simulink model "test_p"  (R2017b)
settings: Solver=VariableStepAuto  StartTime=0.0  StopTime=10.0  RelTol=1e-3
libraries: arduinolib x12
settings Model: Creator=HRUSHIKESH  LastModifiedBy=HRUSHIKESH

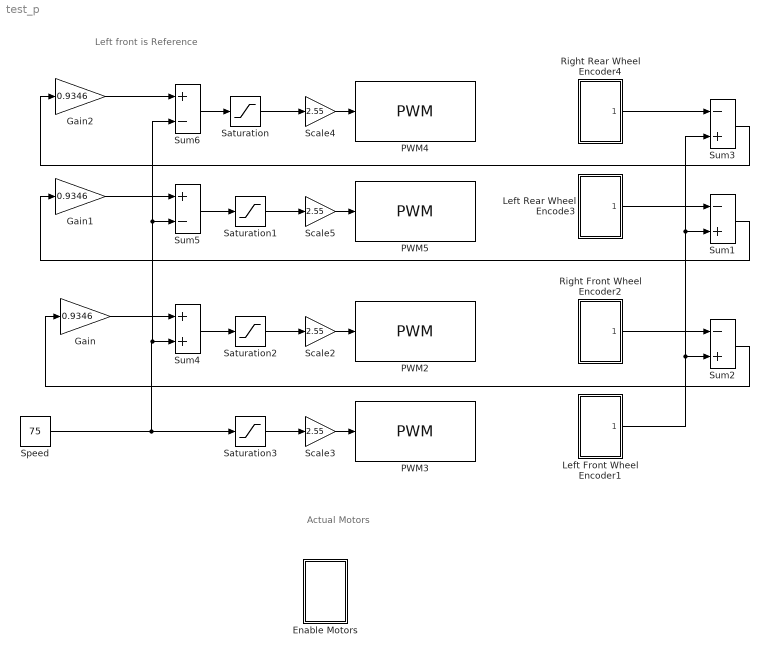
== system test_p ==
  note: Left front is Reference
  note: Actual
      | Motors
  Enable Motors : Subsystem
  Gain : Gain  Gain=0.9346  ParamDataTypeStr=single
  Gain1 : Gain  Gain=0.9346  ParamDataTypeStr=single
  Gain2 : Gain  Gain=0.9346  ParamDataTypeStr=single
  Left Front Wheel Encoder1 : Subsystem
  Left Rear Wheel Encode3 : Subsystem
  PWM2 : arduinolib/PWM  pinNumber=10  blockPlatform=arduino
  PWM3 : arduinolib/PWM  pinNumber=11  blockPlatform=arduino
  PWM4 : arduinolib/PWM  pinNumber=6  blockPlatform=arduino
  PWM5 : arduinolib/PWM  pinNumber=9  blockPlatform=arduino
  Right Front Wheel Encoder2 : Subsystem
  Right Rear Wheel Encoder4 : Subsystem
  Saturation{,1..3} (4 alike) : Saturate  UpperLimit=100  LowerLimit=0
      settings: AttributesFormatString=max = %<UpperLimit>\nmin = %<LowerLimit>
  Scale{2..5} (4 alike) : Gain  Gain=2.55
  Speed : Constant  Value=75  OutMin=0  OutMax=100  OutDataTypeStr=single  SampleTime=0.001
  Sum1 : Sum  Inputs=-+  OutDataTypeStr=Inherit: Same as first input
  Sum2 : Sum  Inputs=-+  OutDataTypeStr=Inherit: Same as first input
  Sum3 : Sum  Inputs=-+  OutDataTypeStr=Inherit: Same as first input
  Sum4 : Sum  OutDataTypeStr=Inherit: Same as first input
  Sum5 : Sum  Inputs=+-  OutDataTypeStr=Inherit: Same as first input
  Sum6 : Sum  Inputs=+-  OutDataTypeStr=Inherit: Same as first input
  wires:
  Scale2/1 -> PWM2/1
  Scale3/1 -> PWM3/1
  Right Rear Wheel Encoder4/1(Encoder) -> Sum3/1
  Scale4/1 -> PWM4/1
  Scale5/1 -> PWM5/1
  Sum3/1 -> Gain2/1
  Right Front Wheel Encoder2/1(Encoder) -> Sum2/1
  Left Rear Wheel Encode3/1(Encoder) -> Sum1/1
  Left Front Wheel Encoder1/1(Encoder) -> Sum3/2, Sum1/2, Sum2/2
  Saturation/1 -> Scale4/1
  Saturation1/1 -> Scale5/1
  Saturation2/1 -> Scale2/1
  Saturation3/1 -> Scale3/1
  Sum1/1 -> Gain1/1
  Sum2/1 -> Gain/1
  Sum6/1 -> Saturation/1
  Sum5/1 -> Saturation1/1
  Sum4/1 -> Saturation2/1
  Speed/1 -> Sum5/2, Sum6/2, Sum4/2, Saturation3/1
  Gain/1 -> Sum4/1
  Gain2/1 -> Sum6/1
  Gain1/1 -> Sum5/1

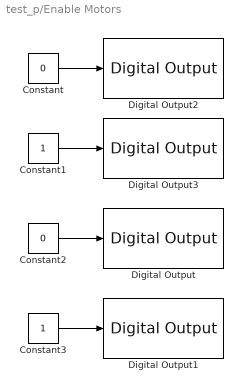
== system test_p/Enable Motors ==
  Constant : Constant  Value=0  OutDataTypeStr=boolean
  Constant1 : Constant  OutDataTypeStr=boolean
  Constant2 : Constant  Value=0  OutDataTypeStr=boolean
  Constant3 : Constant  OutDataTypeStr=boolean
  Digital Output : arduinolib/Digital Output  pinNumber=a1  blockPlatform=arduino
  Digital Output1 : arduinolib/Digital Output  pinNumber=a0  blockPlatform=arduino
  Digital Output2 : arduinolib/Digital Output  pinNumber=a3  blockPlatform=arduino
  Digital Output3 : arduinolib/Digital Output  pinNumber=a2  blockPlatform=arduino
  wires:
  Constant3/1 -> Digital Output1/1
  Constant2/1 -> Digital Output/1
  Constant/1 -> Digital Output2/1
  Constant1/1 -> Digital Output3/1

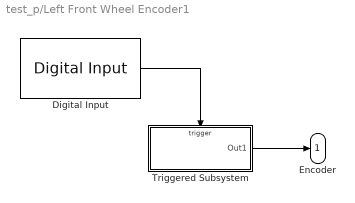
== system test_p/Left Front Wheel Encoder1 ==
  Digital Input : arduinolib/Digital Input  pinNumber=1  sampleTime=0.001  blockPlatform=arduino
      settings: SourceProductName=Simulink Support Package for Arduino Hardware
  Triggered Subsystem : Subsystem  TreatAsAtomicUnit=on
  Encoder : Outport
  wires:
  Triggered Subsystem/1(Out1) -> Encoder/1
  Digital Input/1 -> Triggered Subsystem/Trigger

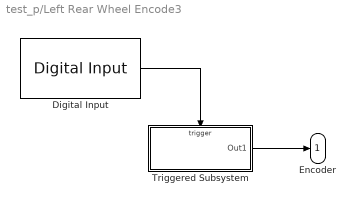
== system test_p/Left Rear Wheel Encode3 ==
  Digital Input : arduinolib/Digital Input  pinNumber=3  sampleTime=0.001  blockPlatform=arduino
      settings: SourceProductName=Simulink Support Package for Arduino Hardware
  Triggered Subsystem : Subsystem  TreatAsAtomicUnit=on
  Encoder : Outport
  wires:
  Triggered Subsystem/1(Out1) -> Encoder/1
  Digital Input/1 -> Triggered Subsystem/Trigger

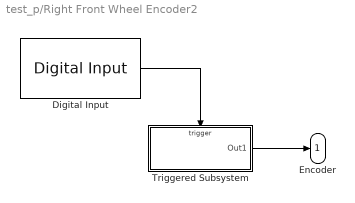
== system test_p/Right Front Wheel Encoder2 ==
  Digital Input : arduinolib/Digital Input  pinNumber=2  sampleTime=0.001  blockPlatform=arduino
      settings: SourceProductName=Simulink Support Package for Arduino Hardware
  Triggered Subsystem : Subsystem  TreatAsAtomicUnit=on
  Encoder : Outport
  wires:
  Digital Input/1 -> Triggered Subsystem/Trigger
  Triggered Subsystem/1(Out1) -> Encoder/1

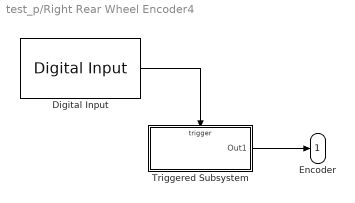
== system test_p/Right Rear Wheel Encoder4 ==
  Digital Input : arduinolib/Digital Input  pinNumber=4  sampleTime=0.001  blockPlatform=arduino
      settings: SourceProductName=Simulink Support Package for Arduino Hardware
  Triggered Subsystem : Subsystem  TreatAsAtomicUnit=on
  Encoder : Outport
  wires:
  Digital Input/1 -> Triggered Subsystem/Trigger
  Triggered Subsystem/1(Out1) -> Encoder/1

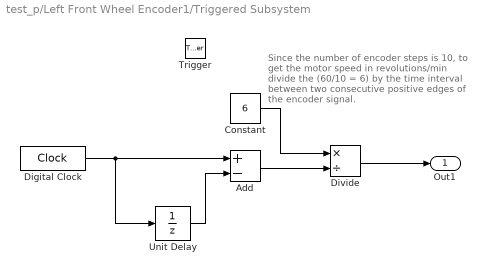
== system test_p/Left Front Wheel Encoder1/Triggered Subsystem ==
  note: Since the number of encoder steps is 10,
      | to get the motor speed in revolutions/min
      | divide the (60/10 = 6) by the time interval
      | between two consecutive positive edges
      | of the encoder signal.
  Trigger : TriggerPort  VariantControl=Variant
  Add : Sum  Inputs=+-
  Constant : Constant  Value=6
  Digital Clock : DigitalClock  SampleTime=-1
  Divide : Product  Inputs=*/  OutDataTypeStr=int32
  Unit Delay : UnitDelay  SampleTime=-1
  Out1 : Outport
  wires:
  Digital Clock/1 -> Add/1, Unit Delay/1
  Unit Delay/1 -> Add/2
  Add/1 -> Divide/2
  Divide/1 -> Out1/1
  Constant/1 -> Divide/1

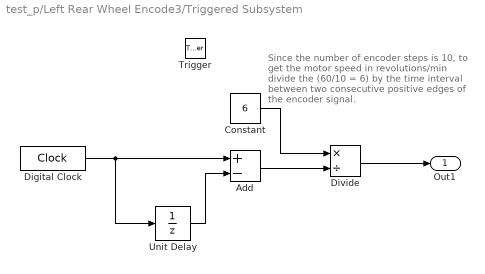
== system test_p/Left Rear Wheel Encode3/Triggered Subsystem ==
  note: Since the number of encoder steps is 10,
      | to get the motor speed in revolutions/min
      | divide the (60/10 = 6) by the time interval
      | between two consecutive positive edges
      | of the encoder signal.
  Trigger : TriggerPort  VariantControl=Variant
  Add : Sum  Inputs=+-
  Constant : Constant  Value=6
  Digital Clock : DigitalClock  SampleTime=-1
  Divide : Product  Inputs=*/  OutDataTypeStr=int32
  Unit Delay : UnitDelay  SampleTime=-1
  Out1 : Outport
  wires:
  Digital Clock/1 -> Add/1, Unit Delay/1
  Unit Delay/1 -> Add/2
  Add/1 -> Divide/2
  Divide/1 -> Out1/1
  Constant/1 -> Divide/1

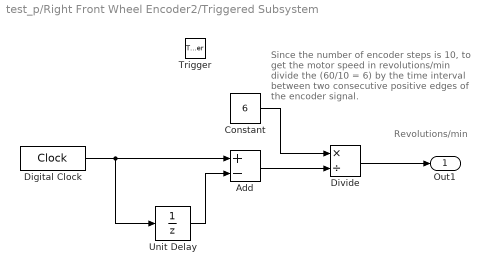
== system test_p/Right Front Wheel Encoder2/Triggered Subsystem ==
  note: Revolutions/min
  note: Since the number of encoder steps is 10,
      | to get the motor speed in revolutions/min
      | divide the (60/10 = 6) by the time interval
      | between two consecutive positive edges
      | of the encoder signal.
  Trigger : TriggerPort  VariantControl=Variant
  Add : Sum  Inputs=+-
  Constant : Constant  Value=6
  Digital Clock : DigitalClock  SampleTime=-1
  Divide : Product  Inputs=*/  OutDataTypeStr=int32
  Unit Delay : UnitDelay  SampleTime=-1
  Out1 : Outport
  wires:
  Constant/1 -> Divide/1
  Divide/1 -> Out1/1
  Add/1 -> Divide/2
  Unit Delay/1 -> Add/2
  Digital Clock/1 -> Unit Delay/1, Add/1

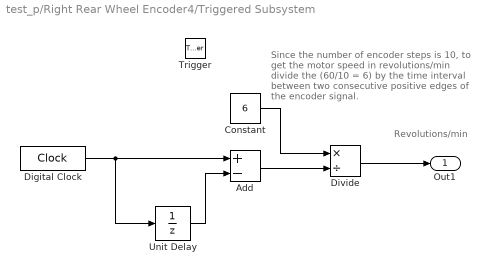
== system test_p/Right Rear Wheel Encoder4/Triggered Subsystem ==
  note: Revolutions/min
  note: Since the number of encoder steps is 10,
      | to get the motor speed in revolutions/min
      | divide the (60/10 = 6) by the time interval
      | between two consecutive positive edges
      | of the encoder signal.
  Trigger : TriggerPort  VariantControl=Variant
  Add : Sum  Inputs=+-
  Constant : Constant  Value=6
  Digital Clock : DigitalClock  SampleTime=-1
  Divide : Product  Inputs=*/  OutDataTypeStr=int32
  Unit Delay : UnitDelay  SampleTime=-1
  Out1 : Outport
  wires:
  Constant/1 -> Divide/1
  Divide/1 -> Out1/1
  Add/1 -> Divide/2
  Unit Delay/1 -> Add/2
  Digital Clock/1 -> Unit Delay/1, Add/1
